simulink model "CasterBicycleModel_Group1_Zhicun_Andreas"  (R2022a)
settings: Solver=VariableStepAuto  StartTime=0.0  StopTime=10.0  RelTol=1e-3  EnableMultiTasking=on
undefined symbols (not defined in the file or in its folder): vehicleData
settings Model: Creator=parp  LastModifiedBy=tanzc
settings SolverCC: AlgebraicLoopSolver=TrustRegion
settings DataIOCC: LimitDataPoints=on  ReturnWorkspaceOutputs=off
settings OptimizationCC: LifeSpan=inf
settings DebuggingCC: UnconnectedInputMsg=warning  UnconnectedOutputMsg=warning  UnconnectedLineMsg=warning  AllowSymbolicDim=off  SFUnexpectedBacktrackingDiag=warning  SFNoUnconditionalDefaultTransitionDiag=warning  SFExecutionAtInitializationDiag=none  SFMachineParentedDataDiag=warning  ArithmeticOperatorsInVariantConditions=warning
settings ModelReferenceCC: PropagateSignalLabelsOutOfModel=off
settings SFSimCC: SimUseLocalCustomCode=off  CustomCodeUndefinedFunction=UseInterfaceOnly
settings RTWCC: RTWUseLocalCustomCode=off
settings CodeAppCC: StateflowObjectComments=on
settings GRTTargetCC: TargetLangStandard=C89/C90 (ANSI)
settings ConfigComp: CovMetricSettings=dw  CovSaveCumulativeToWorkspaceVar=on  CovSaveSingleToWorkspaceVar=on  CovExternalEMLEnable=off

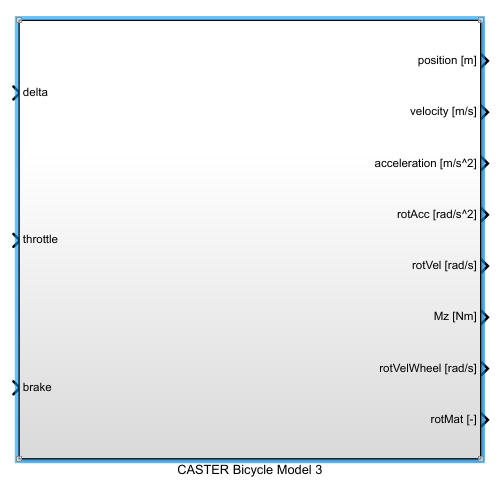
[thumbnail: Simulink's stored preview of the top-level diagram]
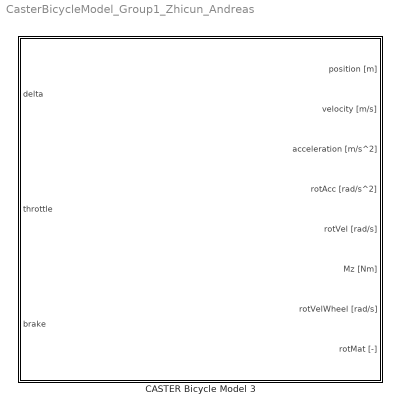
== system CasterBicycleModel_Group1_Zhicun_Andreas ==
  CASTER Bicycle Model 3 : Subsystem

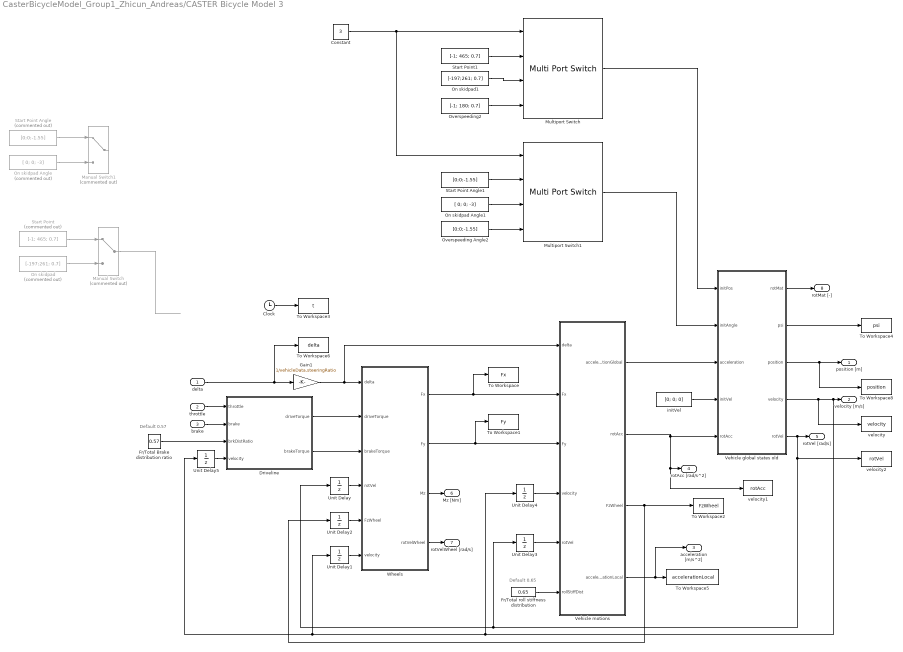
== system CasterBicycleModel_Group1_Zhicun_Andreas/CASTER Bicycle Model 3 ==
  note: Default 0.65
  note: Default 0.57
  delta : Inport
  throttle : Inport  Port=2
  brake : Inport  Port=3
  Clock : Clock
  Constant : Constant  Value=3
  Driveline : Subsystem
  Fr/Total Brake distribution ratio : Constant  Value=0.57  VectorParams1D=off
  Fr/Total roll stiffness distribution : Constant  Value=0.65
  Gain1 : Gain  Gain=1/vehicleData.steeringRatio
  Manual Switch : ManualSwitch  Commented=on
  Manual Switch1 : ManualSwitch  Commented=on
  Multiport Switch : MultiPortSwitch  SaturateOnIntegerOverflow=off  InputSameDT=off
  Multiport Switch1 : MultiPortSwitch  SaturateOnIntegerOverflow=off  InputSameDT=off
  On skidpad : Constant  Commented=on  Value=[-197;261; 0.7]
  On skidpad Angle : Constant  Commented=on  Value=[ 0; 0; -3]
  On skidpad Angle1 : Constant  Value=[ 0; 0; -3]
  On skidpad1 : Constant  Value=[-197;261; 0.7]
  Overspeeding Angle2 : Constant  Value=[0;0;-1.55]
  Overspeeding2 : Constant  Value=[-1; 180; 0.7]
  Start Point : Constant  Commented=on  Value=[-1; 465; 0.7]
  Start Point Angle : Constant  Commented=on  Value=[0;0;-1.55]
  Start Point Angle1 : Constant  Value=[0;0;-1.55]
  Start Point1 : Constant  Value=[-1; 465; 0.7]
  To Workspace : ToWorkspace  VariableName=Fx  SampleTime=-1
  To Workspace1 : ToWorkspace  VariableName=Fy  SampleTime=-1
  To Workspace2 : ToWorkspace  VariableName=FzWheel  SampleTime=-1
  To Workspace3 : ToWorkspace  VariableName=t  SampleTime=-1
  To Workspace4 : ToWorkspace  VariableName=psi  SampleTime=-1
  To Workspace5 : ToWorkspace  VariableName=accelerationLocal  SampleTime=-1
  To Workspace6 : ToWorkspace  VariableName=delta  SampleTime=-1
  To Workspace8 : ToWorkspace  VariableName=position  SampleTime=-1
  Unit Delay{,1..5} (6 alike) : UnitDelay  SampleTime=-1  HasFrameUpgradeWarning=on
  Vehicle global states old : Subsystem
  Vehicle motions : Subsystem
  Wheels : Subsystem
  initVel : Constant  Value=[0; 0; 0]
  velocity : ToWorkspace  VariableName=velocity  SampleTime=-1
  velocity1 : ToWorkspace  VariableName=rotAcc  SampleTime=-1
  velocity2 : ToWorkspace  VariableName=rotVel  SampleTime=-1
  position [m] : Outport
  velocity [m/s] : Outport  Port=2
  acceleration [m/s^2] : Outport  Port=3
  rotAcc [rad/s^2] : Outport  Port=4
  rotVel [rad/s] : Outport  Port=5
  Mz [Nm] : Outport  Port=6
  rotVelWheel [rad/s] : Outport  Port=7
  rotMat [-] : Outport  Port=8
  wires:
  throttle/1 -> Driveline/1(throttle)
  brake/1 -> Driveline/2(brake)
  delta/1 -> To Workspace6/1, Gain1/1
  Unit Delay4/1 -> Vehicle motions/4(velocity)
  Driveline/2(brakeTorque) -> Wheels/3(brakeTorque)
  Driveline/1(driveTorque) -> Wheels/2(driveTorque)
  Wheels/1(Fx) -> Vehicle motions/2(Fx), To Workspace/1
  Wheels/2(Fy) -> Vehicle motions/3(Fy), To Workspace1/1
  Unit Delay3/1 -> Vehicle motions/5(rotVel)
  Vehicle motions/3(FzWheel) -> Unit Delay2/1, To Workspace2/1
  Unit Delay2/1 -> Wheels/5(FzWheel)
  Fr/Total Brake distribution ratio/1 -> Driveline/3(brkDistRatio)
  Fr/Total roll stiffness distribution/1 -> Vehicle motions/6(rollStiffDist)
  Unit Delay/1 -> Wheels/4(rotVel)
  Unit Delay1/1 -> Wheels/6(velocity)
  Wheels/4(rotVelWheel) -> rotVelWheel [rad/s]/1
  Wheels/3(Mz) -> Mz [Nm]/1
  Vehicle motions/2(rotAcc) -> rotAcc [rad/s^2]/1, velocity1/1, Vehicle global states old/5(rotAcc)
  initVel/1 -> Vehicle global states old/4(initVel)
  Vehicle global states old/2(psi) -> To Workspace4/1
  Vehicle global states old/1(rotMat) -> rotMat [-]/1
  Vehicle global states old/5(rotVel) -> Unit Delay3/1, Unit Delay/1, velocity2/1, rotVel [rad/s]/1
  Vehicle global states old/4(velocity) -> velocity/1, Unit Delay4/1, Unit Delay5/1, Unit Delay1/1, velocity [m/s]/1
  Unit Delay5/1 -> Driveline/4(velocity)
  Gain1/1 -> Vehicle motions/1(delta), Wheels/1(delta)
  Clock/1 -> To Workspace3/1
  Vehicle global states old/3(position) -> To Workspace8/1, position [m]/1
  Vehicle motions/1(accelerationGlobal) -> Vehicle global states old/3(acceleration)
  Vehicle motions/4(accelerationLocal) -> acceleration [m/s^2]/1, To Workspace5/1
  Multiport Switch1/1 -> Vehicle global states old/2(initAngle)
  Start Point Angle/1 -> Manual Switch1/1
  On skidpad Angle/1 -> Manual Switch1/2
  Start Point1/1 -> Multiport Switch/2
  On skidpad1/1 -> Multiport Switch/3
  Overspeeding2/1 -> Multiport Switch/4
  Multiport Switch/1 -> Vehicle global states old/1(initPos)
  Manual Switch/1 -> ?
  Start Point/1 -> Manual Switch/1
  On skidpad/1 -> Manual Switch/2
  Constant/1 -> Multiport Switch1/1, Multiport Switch/1
  Start Point Angle1/1 -> Multiport Switch1/2
  On skidpad Angle1/1 -> Multiport Switch1/3
  Overspeeding Angle2/1 -> Multiport Switch1/4

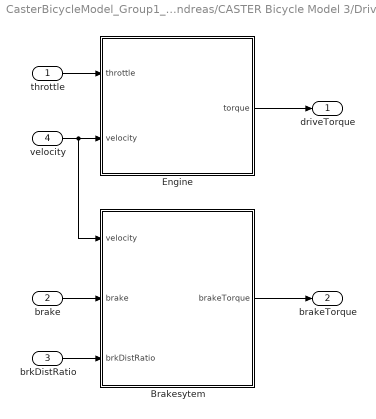
== system CasterBicycleModel_Group1_Zhicun_Andreas/CASTER Bicycle Model 3/Driveline ==
  throttle : Inport
  brake : Inport  Port=2
  brkDistRatio : Inport  Port=3
  velocity : Inport  Port=4
  Brakesytem : MATLAB Function  TreatAsAtomicUnit=on
  Engine : MATLAB Function  TreatAsAtomicUnit=on
  driveTorque : Outport
  brakeTorque : Outport  Port=2
  wires:
  throttle/1 -> Engine/1(throttle)
  brake/1 -> Brakesytem/2(brake)
  Engine/1(torque) -> driveTorque/1
  Brakesytem/1(brakeTorque) -> brakeTorque/1
  brkDistRatio/1 -> Brakesytem/3(brkDistRatio)
  velocity/1 -> Brakesytem/1(velocity), Engine/2(velocity)

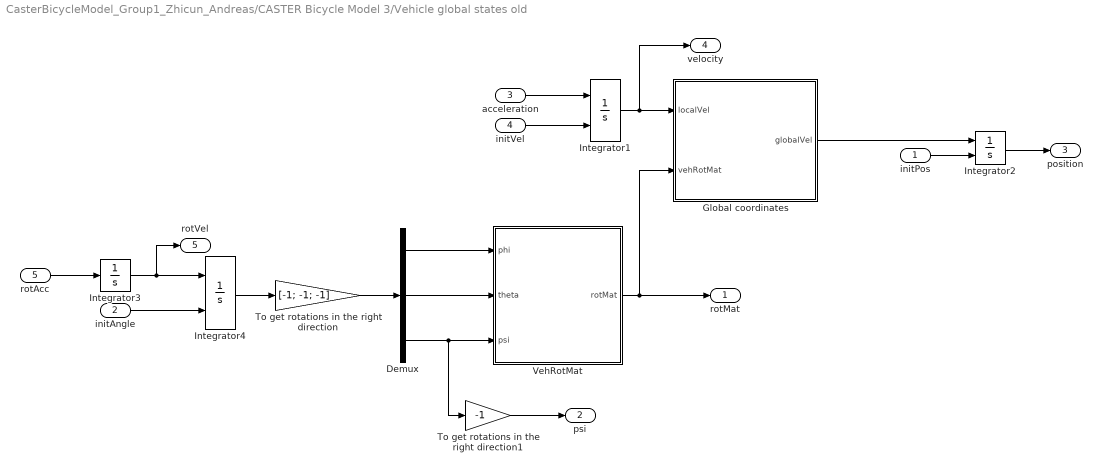
== system CasterBicycleModel_Group1_Zhicun_Andreas/CASTER Bicycle Model 3/Vehicle global states old ==
  initPos : Inport
  initAngle : Inport  Port=2
  acceleration : Inport  Port=3
  initVel : Inport  Port=4
  rotAcc : Inport  Port=5
  Demux : Demux  Outputs=3
  Global coordinates : MATLAB Function  TreatAsAtomicUnit=on
  Integrator1 : Integrator  InitialConditionSource=external  InitialCondition=[0 0 0]  LimitOutput=on  UpperSaturationLimit=90/3.6
  Integrator2 : Integrator  InitialConditionSource=external  InitialCondition=[0; 0; 2]
  Integrator3 : Integrator  InitialCondition=[0 0 0]  UpperSaturationLimit=200  LowerSaturationLimit=-200
  Integrator4 : Integrator  InitialConditionSource=external  InitialCondition=[0 0 0]  UpperSaturationLimit=200  LowerSaturationLimit=-200
  To get rotations in the right direction : Gain  Gain=[-1; -1; -1]
  To get rotations in the right direction1 : Gain  Gain=-1
  VehRotMat : MATLAB Function  TreatAsAtomicUnit=on
  rotMat : Outport
  psi : Outport  Port=2
  position : Outport  Port=3
  velocity : Outport  Port=4
  rotVel : Outport  Port=5
  wires:
  acceleration/1 -> Integrator1/1
  Integrator3/1 -> Integrator4/1, rotVel/1
  Demux/2 -> VehRotMat/2(theta)
  Demux/3 -> To get rotations in the right direction1/1, VehRotMat/3(psi)
  Global coordinates/1(globalVel) -> Integrator2/1
  Integrator1/1 -> Global coordinates/1(localVel), velocity/1
  rotAcc/1 -> Integrator3/1
  Demux/1 -> VehRotMat/1(phi)
  To get rotations in the right direction/1 -> Demux/1
  Integrator4/1 -> To get rotations in the right direction/1
  Integrator2/1 -> position/1
  VehRotMat/1(rotMat) -> Global coordinates/2(vehRotMat), rotMat/1
  initVel/1 -> Integrator1/2
  To get rotations in the right direction1/1 -> psi/1
  initPos/1 -> Integrator2/2
  initAngle/1 -> Integrator4/2

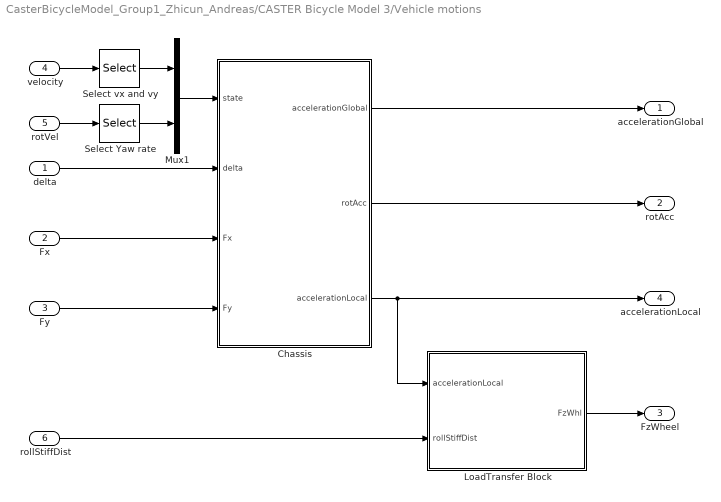
== system CasterBicycleModel_Group1_Zhicun_Andreas/CASTER Bicycle Model 3/Vehicle motions ==
  delta : Inport
  Fx : Inport  Port=2
  Fy : Inport  Port=3
  velocity : Inport  Port=4
  rotVel : Inport  Port=5
  rollStiffDist : Inport  Port=6
  Chassis : MATLAB Function  TreatAsAtomicUnit=on
  LoadTransfer Block : MATLAB Function  TreatAsAtomicUnit=on
  Mux1 : Mux  Inputs=2
  Select Yaw rate : Selector  InputPortWidth=3  IndexOptions=Index vector (dialog)  Indices=[3]  OutputSizes=1
  Select vx and vy : Selector  InputPortWidth=3  IndexOptions=Index vector (dialog)  Indices=[1 2]  OutputSizes=1
  accelerationGlobal : Outport
  rotAcc : Outport  Port=2
  FzWheel : Outport  Port=3
  accelerationLocal : Outport  Port=4
  wires:
  LoadTransfer Block/1(FzWhl) -> FzWheel/1
  Select vx and vy/1 -> Mux1/1
  Select Yaw rate/1 -> Mux1/2
  Mux1/1 -> Chassis/1(state)
  velocity/1 -> Select vx and vy/1
  rotVel/1 -> Select Yaw rate/1
  delta/1 -> Chassis/2(delta)
  Fx/1 -> Chassis/3(Fx)
  Fy/1 -> Chassis/4(Fy)
  Chassis/1(accelerationGlobal) -> accelerationGlobal/1
  Chassis/2(rotAcc) -> rotAcc/1
  Chassis/3(accelerationLocal) -> LoadTransfer Block/1(accelerationLocal), accelerationLocal/1
  rollStiffDist/1 -> LoadTransfer Block/2(rollStiffDist)

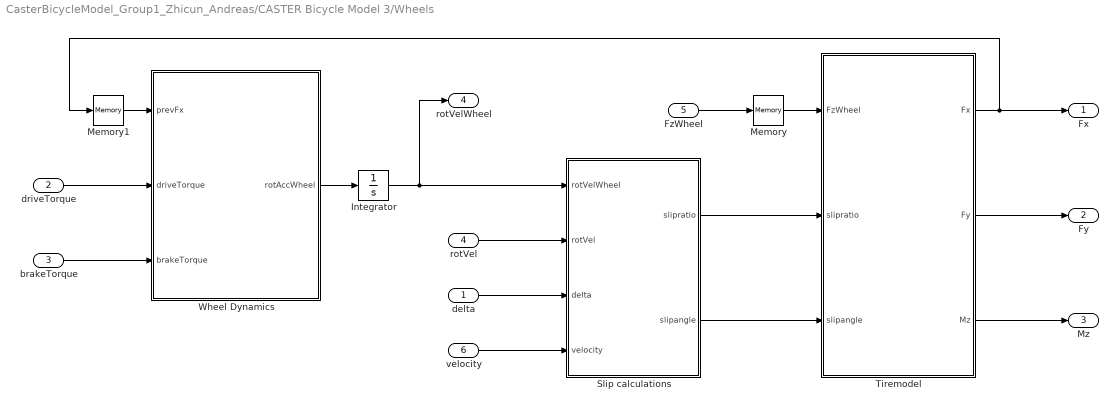
== system CasterBicycleModel_Group1_Zhicun_Andreas/CASTER Bicycle Model 3/Wheels ==
  delta : Inport
  driveTorque : Inport  Port=2
  brakeTorque : Inport  Port=3
  rotVel : Inport  Port=4
  FzWheel : Inport  Port=5
  velocity : Inport  Port=6
  Integrator : Integrator  UpperSaturationLimit=20  LowerSaturationLimit=-20
  Memory : Memory  InitialCondition=vehicleData.m*vehicleData.g/4*ones(4,1)
  Memory1 : Memory  InitialCondition=[0; 0]
  Slip calculations : Subsystem
  Tiremodel : Subsystem
  Wheel Dynamics : MATLAB Function  TreatAsAtomicUnit=on
  Fx : Outport
  Fy : Outport  Port=2
  Mz : Outport  Port=3
  rotVelWheel : Outport  Port=4
  wires:
  brakeTorque/1 -> Wheel Dynamics/3(brakeTorque)
  rotVel/1 -> Slip calculations/2(rotVel)
  Slip calculations/1(slipratio) -> Tiremodel/2(slipratio)
  Slip calculations/2(slipangle) -> Tiremodel/3(slipangle)
  Tiremodel/1(Fx) -> Fx/1, Memory1/1
  Tiremodel/2(Fy) -> Fy/1
  FzWheel/1 -> Memory/1
  delta/1 -> Slip calculations/3(delta)
  velocity/1 -> Slip calculations/4(velocity)
  Memory1/1 -> Wheel Dynamics/1(prevFx)
  Memory/1 -> Tiremodel/1(FzWheel)
  Integrator/1 -> Slip calculations/1(rotVelWheel), rotVelWheel/1
  Tiremodel/3(Mz) -> Mz/1
  Wheel Dynamics/1(rotAccWheel) -> Integrator/1
  driveTorque/1 -> Wheel Dynamics/2(driveTorque)

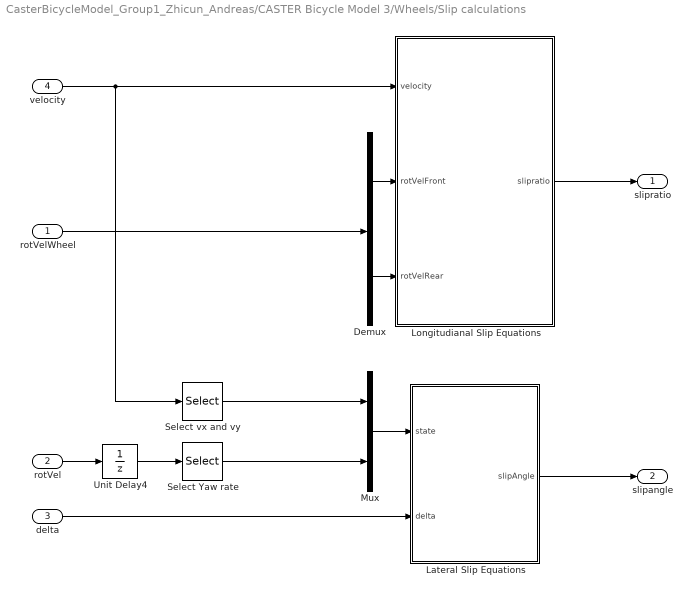
== system CasterBicycleModel_Group1_Zhicun_Andreas/CASTER Bicycle Model 3/Wheels/Slip calculations ==
  rotVelWheel : Inport
  rotVel : Inport  Port=2
  delta : Inport  Port=3
  velocity : Inport  Port=4
  Demux : Demux  Outputs=2
  Lateral Slip Equations : MATLAB Function  TreatAsAtomicUnit=on
  Longitudianal Slip Equations : MATLAB Function  TreatAsAtomicUnit=on
  Mux : Mux  Inputs=2
  Select Yaw rate : Selector  InputPortWidth=3  IndexOptions=Index vector (dialog)  Indices=[3]  OutputSizes=1
  Select vx and vy : Selector  InputPortWidth=3  IndexOptions=Index vector (dialog)  Indices=[1 2]  OutputSizes=1
  Unit Delay4 : UnitDelay  SampleTime=-1  HasFrameUpgradeWarning=on
  slipratio : Outport
  slipangle : Outport  Port=2
  wires:
  velocity/1 -> Select vx and vy/1, Longitudianal Slip Equations/1(velocity)
  rotVelWheel/1 -> Demux/1
  Demux/1 -> Longitudianal Slip Equations/2(rotVelFront)
  Longitudianal Slip Equations/1(slipratio) -> slipratio/1
  Demux/2 -> Longitudianal Slip Equations/3(rotVelRear)
  delta/1 -> Lateral Slip Equations/2(delta)
  rotVel/1 -> Unit Delay4/1
  Select vx and vy/1 -> Mux/1
  Select Yaw rate/1 -> Mux/2
  Mux/1 -> Lateral Slip Equations/1(state)
  Lateral Slip Equations/1(slipAngle) -> slipangle/1
  Unit Delay4/1 -> Select Yaw rate/1

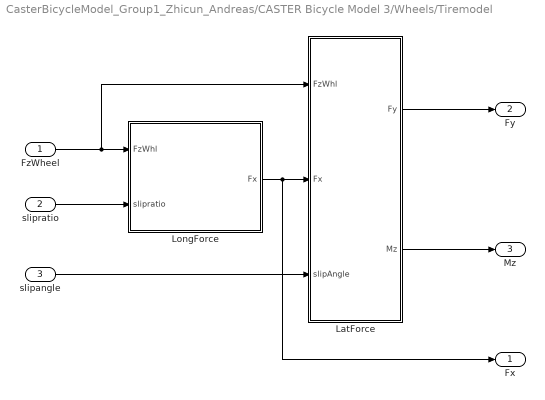
== system CasterBicycleModel_Group1_Zhicun_Andreas/CASTER Bicycle Model 3/Wheels/Tiremodel ==
  FzWheel : Inport
  slipratio : Inport  Port=2
  slipangle : Inport  Port=3
  LatForce : MATLAB Function  TreatAsAtomicUnit=on
  LongForce : MATLAB Function  TreatAsAtomicUnit=on
  Fx : Outport
  Fy : Outport  Port=2
  Mz : Outport  Port=3
  wires:
  FzWheel/1 -> LatForce/1(FzWhl), LongForce/1(FzWhl)
  slipangle/1 -> LatForce/3(slipAngle)
  slipratio/1 -> LongForce/2(slipratio)
  LongForce/1(Fx) -> Fx/1, LatForce/2(Fx)
  LatForce/1(Fy) -> Fy/1
  LatForce/2(Mz) -> Mz/1

== matlab function CasterBicycleModel_Group1_Zhicun_Andreas/CASTER Bicycle Model 3/Wheels/Tiremodel/LongForce ==
  data: FzWhl input; slipratio input; Fx output
function Fx = LongForce(FzWhl,slipratio)
    %   © CASTER / MMF062
    %   Created: 2017-10-01
    % Inputs:
    %   FzWhl     - Normal load on tires [N]
    %   slipratio - Slip ratio [rad]
    % Outputs:
    %   Fx        - A [2x1] vector with axle longitudinal forces [N]
    %
    
    % mu          = 0.8;                                  % Limiting friction corfficient
    % FzWhl       = max(FzWhl,[0;0;0;0]);                 % Make sure normal load on wheel does not become negative
    % FzFrontAxle = FzWhl(1)+FzWhl(2);                    % Front axle normal load
    % FzRearAxle  = FzWhl(3)+FzWhl(4);                    % Rear axle normal load

    % ----- Longitudinal forces -----
    Cx      = 10000*ones(4,1);
    FxFront = -slipratio(1)*(Cx(1)+Cx(2)); 
    FxRear  = -slipratio(2)*(Cx(3)+Cx(4)); 
    % FxFront = min(mu*FzFrontAxle,abs(FxFront))*sign(FxFront);
    % FxRear  = min(mu*FzRearAxle,abs(FxRear))*sign(FxRear);
    Fx      = [FxFront;FxRear];
end

% end of file

== matlab function CasterBicycleModel_Group1_Zhicun_Andreas/CASTER Bicycle Model 3/Wheels/Slip calculations/Lateral Slip Equations ==
  data: state input; slipAngle output; delta input; vehicleData parameter
function slipAngle   = LateralSlip(state,delta,vehicleData) 
    %   © CASTER / MMF062
    %   Created: 2019-11-18
    % Inputs:
    %   state     - State vector
    %   delta     - steering wheel angle [rad]
    % Outputs:
    %   slipangle - A [2x1] vector containing the slipratio(0-1) for each axle [-]
    %
    %%========================DO NOT CHANGE THIS=============================%%
    % ----- Parameters -----
    % State vector
    vx = state(1);
    vy = state(2);
    wz = state(3);
    lf = vehicleData.lf;           % Distance of CoG from front axle
    lr = vehicleData.lr;           % Distance of CoG from rear axle
    % Preventing vx from being zero 
    vx = max(abs(vx),3);

    %%=======================================================================%%
    % Slip equations
    alphaf    = atan2(vy + lf*wz,vx) - delta;   %  Front lateral tire slip 
    alphar    = atan2(vy - lr*wz,vx);          %  Rear lateral tire slip
    
    slipAngle = [alphaf; alphar];  % Slip angle vector
    %%=======================================================================%%

end

% end of file

== matlab function CasterBicycleModel_Group1_Zhicun_Andreas/CASTER Bicycle Model 3/Vehicle motions/LoadTransfer Block ==
  data: accelerationLocal input; rollStiffDist input; vehicleData parameter; FzWhl output
function FzWhl  = RollModel(accelerationLocal,rollStiffDist,vehicleData)
    %   © CASTER / MMF062
    %   Created: 2019-11-18
    % Inputs: 
    %   accelerationLocal - vector of vehicle loacl acceleration [ax; ay; az;]
    %   rollStiffDist     - Roll stiffness distribution 0-1 on the front axle [-]
    % Outputs: 
    %   FzWhl             - vector of tyre normal forces [N]
    %
    % ----- Parameters -----
    
    %%========================DO NOT CHANGE THIS=============================%%
    h       = vehicleData.h;            % Center of gravity height
    g       = vehicleData.g;            % Acceleration due to gravity
    m       = vehicleData.m;            % Mass of vehicle
    cRoll   = vehicleData.cw;           % Total roll stiffness
    h1      = vehicleData.hrcf;         % Front roll center height
    h2      = vehicleData.hrcr;         % Rear roll center height
    L       = vehicleData.L;            % Wheelbase
    lf      = vehicleData.lf;           % Distance of CoG from front axle
    lr      = vehicleData.lr;           % Distance of CoG from rear axle
    dh      = h-(h1*lr+h2*lf)/L;        % Height of CoG from roll axis
    w       = vehicleData.w;            % Vehicle track width
    cfRoll  = cRoll*rollStiffDist;      % Front roll stiffness
    crRoll  = cRoll-cfRoll;             % Rear roll stiffness

    %%=======================================================================%%
    % Longitudinal and lateral acceleration
    ax      = accelerationLocal(1); 
    ay      = accelerationLocal(2);
    
    % Longitudinal load transfer (should be modified by students for tasks 3 and 4.)
    deltaFflzLong = -m*ax*h/L/2;                      % Front left
    deltaFfrzLong = -m*ax*h/L/2;                      % Front right
    deltaFrlzLong =  m*ax*h/L/2;                      % Rear left
    deltaFrrzLong =  m*ax*h/L/2;                      % Rear right  

    % Lateral load transfer (should be modified by students for tasks 3 and 4.)
    deltaFflzLat  = -ay*((h1*lr)/(L*w)+(dh/w)*cfRoll/cRoll)*m;    % Front left
    deltaFfrzLat  =  ay*((h1*lr)/(L*w)+(dh/w)*cfRoll/cRoll)*m;    % Front right
    deltaFrlzLat  = -ay*((h2*lf)/(L*w)+(dh/w)*crRoll/cRoll)*m;    % Rear left
    deltaFrrzLat  =  ay*((h2*lf)/(L*w)+(dh/w)*crRoll/cRoll)*m;    % Rear right
    %%=======================================================================%%

    % Collecting longitudinal and lateral load transfers
    deltaFzLong   = [deltaFflzLong; deltaFfrzLong; deltaFrlzLong; deltaFrrzLong];
    deltaFzLat    = [deltaFflzLat; deltaFfrzLat; deltaFrlzLat; deltaFrrzLat];

    % Total load transfer
    dFz           = deltaFzLong+deltaFzLat;
    FzStatic      = m*g/2/L*[lr; lr; lf; lf];
    FzWhl         = FzStatic+dFz;
    
    %%=======================FOR DRIVING SIMULATOR===========================%%
    % Switch off the load transfer if needed.
    % FzWhl         = FzStatic;
    
    %%========================DO NOT CHANGE THIS=============================%%
    % Wheel lift-off scenario. This is not really *handling* wheel lift-off,
    % but rather making sure the simulation does not crash in the event of
    % wheel lift-off. Solution may still be incorrect. Handling wheel lift-off
    % is not straight forward. So this simulation model is not good for cases
    % with excessive or frequent wheel lift-off.
    if any(FzWhl<=0)
        FzWhl(FzWhl<1e-3) = 1e-3;
    end
end

% end of file

== matlab function CasterBicycleModel_Group1_Zhicun_Andreas/CASTER Bicycle Model 3/Wheels/Wheel Dynamics ==
  data: prevFx input; rotAccWheel output; driveTorque input; brakeTorque input; vehicleData parameter
function rotAccWheel   = fcn(prevFx, driveTorque, brakeTorque, vehicleData)
%   © CASTER / Jacob Gustafsson
%   Created: 2016-10-16
% Inputs:
%   prevFx - A [2x1] vector with the previous longitudinal forces acting on each axle [N]
%   driveTorque - A [2x1] vector with drive torques acting on each axle [Nm]
%   brakeTorque - A [2x1] vector with brake torques acting on each axle [Nm]
% Outputs:
%   rotAccWheel - A [2x1] vector containing rotational accelerations for
%   each axle
%
%% ----- Parameters -----
WheelRadius  = vehicleData.R;
WheelInertia = vehicleData.J_Wheel;

%% ----- Rotational acceleration of wheels -----

% Resulting moment acting on the wheel
resMoment = (driveTorque + brakeTorque - prevFx.*WheelRadius);

% The rotational acceleration created by the moment
rotAccWheel= resMoment./WheelInertia/1;

== matlab function CasterBicycleModel_Group1_Zhicun_Andreas/CASTER Bicycle Model 3/Driveline/Brakesytem ==
  data: velocity input; brake input; brakeTorque output; brkDistRatio input
function brakeTorque = brakeSystem(velocity, brake, brkDistRatio)
%   © CASTER / Jacob Gustafsson
%   Created: 2016-10-16
% Inputs:
%   brake - Brake signal 0-1 [-]
%   brkDistRatio - Brake distribution ratio 0-1 for the front axle [-]
%   velocity - vector with vehicle velocities [vx; vy; vz]
% Outputs:
%   brakeTorque - A [4x1] vector containing the brakeTorques acting on each wheel
%
%% ----- Parameters -----
vx = velocity(1);

%% ----- Brake torque -----

totalBrakeTorque = brake * 13000;   % Equal to about 4000 N at full braking
%if vx <=1 && vx >= -1
%    totalBrakeTorque =0;
%end

brakeTorqueFront = -brkDistRatio*totalBrakeTorque*sign(vx);
brakeTorqueRear = -(1-brkDistRatio)*totalBrakeTorque*sign(vx);
brakeTorque = [brakeTorqueFront/2; brakeTorqueRear/2];

== matlab function CasterBicycleModel_Group1_Zhicun_Andreas/CASTER Bicycle Model 3/Driveline/Engine ==
  data: throttle input; velocity input; torque output; vehicleData parameter
function torque  = engine(throttle, velocity, vehicleData)
%   © CASTER / Jacob Gustafsson
%   Created: 2016-10-16
% Inputs:
%   throttle - Throttle signal 0-1 [-]
%   velocity - vector with vehicle velocities [vx; vy; vz]
% Outputs:
%   torque - A [4x1] vector containing the torque och each wheel
%
%% ----- Parameters -----
Pmax = 154e3;                                       % SAAB 9-3 2.0T engine.
Tmax = 300*10;                                      % SAAB 9-3 2.0T engine.

WheelRadius = vehicleData.R;

vx = max(abs(velocity(1)),0.1);

%% ----- Torque -----

%if Pmax/abs(vx)*throttle >= Tmax/WheelRadius    % Limited by maximum torque
    torqueEngine = Tmax*throttle;
%else                        % Limited by maximum power
%    torqueEngine = Pmax*throttle/abs(vx)*WheelRadius; 
%end

% Torque acting on each wheel
torque = [torqueEngine/2; 0];

== matlab function CasterBicycleModel_Group1_Zhicun_Andreas/CASTER Bicycle Model 3/Vehicle global states old/Global coordinates ==
  data: localVel input; globalVel output; vehRotMat input
function globalVel = globalcoordinates(localVel, vehRotMat)
%   © CASTER / Jacob Gustafsson
%   Created: 2016-10-16
% Inputs:
%   localVel - Vehicle velocity in local coordinate system [vx; vy; vz]
%   vehRotMat - Vehicle rotational matrix
% Outputs:
%   globalVel - Vehicle velocity in global coordinate system [vx; vy; vz]
%
%% ----- Translating local to global coordinate system -----

vehRotMat = reshape(vehRotMat, [3 3]);
globalVel = vehRotMat*localVel;

== matlab function CasterBicycleModel_Group1_Zhicun_Andreas/CASTER Bicycle Model 3/Vehicle global states old/VehRotMat ==
  data: phi input; theta input; rotMat output; psi input
function rotMat = VehRotMat(phi, theta, psi)
%   © CASTER / Jacob Gustafsson
%   Created: 2016-10-16
% Inputs:
%   phi - roll angle [rad]
%   theta - pitch angle [rad]
%   psi - yaw angle [rad]
% Outputs:
%   rotMat - Vehicle rotational matrix
%
%% ----- Ratational matrix -----
% From ridig body dynamics course compendium page 52
RotX=[1 0 0; 0 cos(phi) sin(phi); 0 -sin(phi) cos(phi)];
RotY=[cos(theta) 0 -sin(theta); 0 1 0; sin(theta) 0 cos(theta)];
RotZ=[cos(psi) sin(psi) 0; -sin(psi) cos(psi) 0; 0 0 1];

rotMat=reshape(RotZ*RotY*RotX, 9, 1);

== matlab function CasterBicycleModel_Group1_Zhicun_Andreas/CASTER Bicycle Model 3/Vehicle motions/Chassis ==
  data: state input; accelerationGlobal output; rotAcc output; delta input; Fx input; Fy input; accelerationLocal output; vehicleData parameter
function [accelerationGlobal,rotAcc,accelerationLocal] = VehDynModel(state,delta,Fx,Fy,vehicleData)
    %   © CASTER / MMF062
    %   Created: 2019-11-18
    % Inputs:
    %   state  - state vector
    %   delta  - steering wheel angle [rad]
    %   Fx     - Vector of forces from the wheels in x-direction
    %   Fy     - Vector of forces from the wheels in y-direction
    % Outputs: 
    %   accelerationGlobal  - global vehicle acceleration
    %                         [vxDot; vyDot; vzDot]
    %   rotAcc              - vector of vehicle rotational accelerations
    %                         [wx; wy; wz]
    %   accelerationLocal   - local vehicle acceleration 
    %                         [ax; ay; az]
    %
    % ----- Parameters -----
    %%========================DO NOT CHANGE THIS=============================%%
    m         = vehicleData.m;            % Mass of vehicle
    J         = vehicleData.J;
    lf        = vehicleData.lf;           % Distance of CoG from front axle
    lr        = vehicleData.lr;           % Distance of CoG from rear axle

    % State vector
    vx        = state(1);
    vy        = state(2);
    wz        = state(3);
    
    %%=======================================================================%%
    % Equations of motion

    vxDot     = (Fx(1)*cos(delta) - Fy(1)*sin(delta) + Fx(2))/m + wz*vy;       % Derivative of longtidunial velocity
    vyDot     = (Fx(1)*sin(delta) + Fy(1)*cos(delta) + Fy(2))/m - wz*vx;       % Derivative of lateral velocity
    wzDot     = ((Fx(1)*sin(delta) + Fy(1)*cos(delta))*lf - Fy(2)*lr)/J;       % Derivative of yaw rotational velocity
    
    %%========================DO NOT CHANGE THIS=============================%%
    vzDot     = 0;
    wxDot     = 0;
    wyDot     = 0;
      

    % Accelerations
    accelerationGlobal = [vxDot;vyDot;vzDot];
    ax                 = vxDot-wz*vy; 
    ay                 = vyDot+wz*vx;
    az                 = 0;
    accelerationLocal  = [ax;ay;az];

    % Rotational accelerations
    rotAcc             = [wxDot;wyDot;wzDot];
    %%=======================================================================%%
end

% end of file

== matlab function CasterBicycleModel_Group1_Zhicun_Andreas/CASTER Bicycle Model 3/Wheels/Tiremodel/LatForce ==
  data: FzWhl input; Fx input; slipAngle input; Fy output; vehicleData parameter; Mz output
function [Fy,Mz]  = LatForce(FzWhl,Fx,slipAngle,vehicleData)
%#codegen
    %   © CASTER / MMF062
    %   Created: 2019-11-18
    % Inputs:
    %   FzWhl      - Normal load on tires [N]
    %   Fx         - Longitudinal force vector [N]
    %   slipAngle  - Slip angle vector [rad]
    % Outputs:
    %   Fy         - A [2x1] vector with axle lateral forces [N]
    %   Mz         - Dummy value for StrWhlTrq [Nm]
    %
    %%========================DO NOT CHANGE THIS=============================%%
    c0          = vehicleData.c0;                       % Tyre stiffness parameter
    c1          = vehicleData.c1;                       % Tyre stiffness parameter
    mu          = 0.8;

    FzWhl       = max(FzWhl,[0;0;0;0]);                 % Limit minimum value
    FzFrontAxle = FzWhl(1)+FzWhl(2);                    % Front axle normal load
    FzRearAxle  = FzWhl(3)+FzWhl(4);                    % Rear axle normal load
    FzAxle      = [FzFrontAxle;FzRearAxle];
    %%=======================================================================%%
    
    % Axle stiffness calculation (keep in mind that the tyre data is for one
    % wheel and not an axle)
    maxLatForce = [0;0];
    
    % Fx could have been limited when it is calculated
    if (Fx(1)^2>=(mu*FzFrontAxle)^2)
        Cf             = 1e-3;                             % Solving the numerical problems
        maxLatForce(1) = 0;
    else
        %%=======================================================================%%
        Cf             =  (c0*FzWhl(1) + c1*FzWhl(1)^2) + (c0*FzWhl(2) + c1*FzWhl(2)^2); % Front cornering stiffness
        %%=======================================================================%%
        
        maxLatForce(1) = sqrt((mu*FzAxle(1))^2-Fx(1)^2);   % Friction circle
        
        %%=============================FOR TASK 4================================%%
        % Combined Slip
        Cf             =  Cf * sqrt((mu*FzAxle(1))^2-Fx(1)^2)/(mu*FzAxle(1));
        %%=======================================================================%%
    end
    
    if (Fx(2)^2>=(mu*FzRearAxle)^2)
        Cr             = 1e-3;                             % Solving the numerical problems
        maxLatForce(2) = 0;
    else
        %%=======================================================================%%
        Cr             =  (c0*FzWhl(3) + c1*FzWhl(3)^2) + (c0*FzWhl(4) + c1*FzWhl(4)^2);% Rear cornering stiffness
        %%=======================================================================%%
        
        maxLatForce(2) = sqrt((mu*FzAxle(2))^2-Fx(2)^2);   % Friction circle
        
        %%=============================FOR TASK 4================================%%
        % Combined Slip
        Cr             =  Cr * sqrt((mu*FzAxle(2))^2-Fx(2)^2)/(mu*FzAxle(2));
        %%=======================================================================%%
    end
    
    % Lateral force
    CAxle = [Cf;Cr];
    Fy    =  -CAxle.*tan(slipAngle);
    
    %%========================DO NOT CHANGE THIS=============================%%
    Fy    = min(maxLatForce,abs(Fy)).*sign(Fy);            % Saturation of Fy to sqrt(Fz^2-Fx^2)
    %%=======================================================================%%
    % Self-aligning moment
    A  = -0.001;
    C  = 0.4;
    Mz = A*Fy(1)*C;
    %%=======================================================================%%
end

== matlab function CasterBicycleModel_Group1_Zhicun_Andreas/CASTER Bicycle Model 3/Wheels/Slip calculations/Longitudianal Slip Equations ==
  data: velocity input; rotVelFront input; rotVelRear input; slipratio output; vehicleData parameter
function slipratio = LongitudinalSlipAngles(velocity, rotVelFront, rotVelRear, vehicleData) 
%   © CASTER / Jacob Gustafsson
%   Created: 2016-10-16
% Inputs:
%   velocity - A [3x1] vector with the vehicle speed [m/s]
%   rotVelFront - A [2x1] vector with rotational velocities for the front wheels [rad/s]
%   rotVelFront - A [2x1] vector with rotational velocities for the rear wheels [rad/s]
% Outputs:
%   slipratio - A [4x1] vector containing the slipratio(0-1) for each wheel [-]
%
%% ----- Parameters -----
WheelRadius = vehicleData.R;
vx          = max(abs(velocity(1)),3);

%% ----- Slipratios -----
% Front and rear slip ratio
alphaf    = -(rotVelFront*WheelRadius-vx)/(vx);
% alphaf    = min(abs(alphaf),0.95)*sign(alphaf);
alphar    = -(rotVelRear*WheelRadius-vx)/(vx);
% alphar    = min(abs(alphar),0.95)*sign(alphar);
slipratio = [alphaf; alphar];

% end of file
